simulink model "INS"  (R2018b)
settings: configuration reference "ins_config" (kept outside this file)
values from neighbouring files (symbols this model uses):
  INS_EXPORT = Simulink.Parameter(INS_EXPORT_VALUE)    [base_ins_init.m]    (also in ins_model_init.m)
  INS_PARAM = Simulink.Parameter(INS_PARAM_VALUE)    [base_ins_init.m]    (also in ins_model_init.m)
undefined symbols (not defined in the file or in its folder): DiscIntNeverNeededParam, INS_CONST
libraries: simulink x95, AP_Math x15, Filter x6, Quaternion x2, Rotation x2
(part 4 of 4)

== system INS/Data_Fusion/AHRS/Correct/Att_Correction/Attitude_Correct/Measured_Acc/OpticalFlow_Acc_Observer ==
  OptFlow_vel_O_mDs : Inport
  Enable : EnablePort  StatesWhenEnabling=reset
  Constant : Constant  Value=0  OutDataTypeStr=single
  ContinueLinearObserver : Subsystem  mask{wn=10, ksi=0.707}
      mask prompts: wn "Cut frequency (rad/s)"; ksi "Damping ratio"
  Mux : Mux  Inputs=2
  Reshape : Reshape  OutputDimensionality=Customize  OutputDimensions=[3,1]
  Selector : Selector  InputPortWidth=3  IndexOptions=Index vector (dialog)  Indices=[1 2]  OutputSizes=1
  Terminator : Terminator
  OptFlow_acc_O_mPs2 : Outport
  wires:
  Mux/1 -> Reshape/1
  OptFlow_vel_O_mDs/1 -> Selector/1
  Constant/1 -> Mux/2
  ContinueLinearObserver/2(x2) -> Mux/1
  ContinueLinearObserver/1(x1) -> Terminator/1
  Selector/1 -> ContinueLinearObserver/1(xr)
  Reshape/1 -> OptFlow_acc_O_mPs2/1

== system INS/Data_Fusion/AHRS/Correct/Att_Correction/Attitude_Correct/Measured_Acc/Routing ==
  gps_ob_enable : Inport
  GPS_acc_O_mPs2 : Inport  Port=2
  opt_flow_ob_enable : Inport  Port=3
  opt_flow_acc_O_mPs2 : Inport  Port=4
  GPS_Delay : Constant  Value=250/INS_EXPORT.period  OutDataTypeStr=uint16
  Logical Operator : Logic  Operator=OR  AllPortsSameDT=off  OutDataTypeStr=boolean
  Multiply{,1..3} (4 alike) : Product  OutDataTypeStr=single
  OptFlow_Delay : Constant  Value=50/INS_EXPORT.period  OutDataTypeStr=uint16
  Sum : Sum  Inputs=|++
  Sum1 : Sum  Inputs=|++
  Sum2 : Sum  Inputs=++|
  gravity : Constant  Value=[0;0;-INS_CONST.g]  VectorParams1D=off  OutDataTypeStr=single
  meas_acc_O_mPs2 : Outport
  acc_ob_valid : Outport  Port=2
  acc_delay : Outport  Port=3
  wires:
  gps_ob_enable/1 -> Logical Operator/1, Multiply/1, Multiply2/1
  Multiply2/1 -> Sum1/1
  GPS_Delay/1 -> Multiply2/2
  Multiply/1 -> Sum/1
  GPS_acc_O_mPs2/1 -> Multiply/2
  opt_flow_acc_O_mPs2/1 -> Multiply1/2
  opt_flow_ob_enable/1 -> Multiply1/1, Multiply3/1, Logical Operator/2
  Multiply1/1 -> Sum/2
  Logical Operator/1 -> acc_ob_valid/1
  OptFlow_Delay/1 -> Multiply3/2
  Sum1/1 -> acc_delay/1
  Multiply3/1 -> Sum1/2
  Sum2/1 -> meas_acc_O_mPs2/1
  Sum/1 -> Sum2/2
  gravity/1 -> Sum2/1

== system INS/Data_Fusion/Translation_Filter/CF/Bus_Assignment/Signal_Rounting/Meter_to_LatLon/Zero_Value_Exclusion ==
  u : Inport
  Abs : Abs
  Constant : Constant
  Product : Product  RndMeth=Zero
  Saturation : Saturate  UpperLimit=10e7  LowerLimit=thr
  Sign : Signum
  Switch : Switch  Criteria=u2 ~= 0
  y : Outport
  wires:
  u/1 -> Sign/1, Abs/1
  Abs/1 -> Saturation/1
  Saturation/1 -> Product/1
  Sign/1 -> Switch/2, Switch/1
  Product/1 -> y/1
  Switch/1 -> Product/2
  Constant/1 -> Switch/3

== system INS/Data_Fusion/Translation_Filter/CF/Horizontal_Filter/Correct/GPS_Correct/Holder ==
  in : Inport
  update : Inport  Port=2
  Gain3 : Gain  Gain=INS_CONST.dt  OutDataTypeStr=Inherit: Same as input
  Memory : Memory
  Switch : Switch  Criteria=u2 > Threshold
  out : Outport
  wires:
  update/1 -> Switch/2
  Switch/1 -> Memory/1, Gain3/1
  in/1 -> Switch/1
  Memory/1 -> Switch/3
  Gain3/1 -> out/1

== system INS/Data_Fusion/Translation_Filter/CF/Horizontal_Filter/Correct/GPS_Correct/Measurement ==
  X : Inport
  Processed_Data : Inport  Port=2
  Bus Selector : BusSelector  OutputSignals=Sensor_Meas.GPS_Meas.mue_rad,Sensor_Meas.GPS_Meas.lambda_rad,Init_Condition.WGS84_Ref.WGS84_pos_ref.mue_0_rad,Init_Condition.WGS84_Ref.WGS84_pos_ref.lambda_0_rad,Init_Condition.WGS84_Ref.WGS84_derivatives_ref.dx_dmue_0,Init_Condition.WGS84_Ref.WGS84_derivatives_ref.dy_dlambda_0
  Bus Selector1 : BusSelector  OutputSignals=Sensor_Meas.GPS_Meas.vel_N_mPs,Sensor_Meas.GPS_Meas.vel_E_mPs
  Data Type Conversion : DataTypeConversion  OutDataTypeStr=single
  Multiply : Product
  Mux{,1..4} (5 alike) : Mux  Inputs=2
  Remove_Bias : Subsystem
  Reshape3 : Reshape  OutputDimensionality=Customize  OutputDimensions=[4,1]
  Sum : Sum  Inputs=|+-
  Z : Outport
  bias_update : Outport  Port=2
  wires:
  X/1 -> Remove_Bias/2(X)
  Data Type Conversion/1 -> Remove_Bias/3(xy_meas_m)
  Remove_Bias/2(xy_O_m) -> Mux3/1
  Bus Selector1/2 -> Mux4/2  "<vel_E_mPs>"
  Bus Selector1/1 -> Mux4/1  "<vel_N_mPs>"
  Multiply/1 -> Data Type Conversion/1  "xy"
  Mux2/1 -> Multiply/2
  Sum/1 -> Multiply/1
  Bus Selector/6 -> Mux2/2  "<dy_dlambda_0>"
  Bus Selector/5 -> Mux2/1  "<dx_dmue_0>"
  Mux1/1 -> Sum/2
  Mux/1 -> Sum/1
  Bus Selector/4 -> Mux1/2  "<lambda_0_rad>"
  Bus Selector/3 -> Mux1/1  "<mue_0_rad>"
  Bus Selector/2 -> Mux/2  "<lambda_rad>"
  Bus Selector/1 -> Mux/1  "<mue_rad>"
  Processed_Data/1 -> Bus Selector/1, Bus Selector1/1, Remove_Bias/1(Processed_Data)
  Remove_Bias/1(bias_update) -> bias_update/1
  Mux3/1 -> Reshape3/1
  Reshape3/1 -> Z/1
  Mux4/1 -> Mux3/2

== system INS/Data_Fusion/Translation_Filter/CF/Horizontal_Filter/Correct/GPS_Correct/Observation ==
  X : Inport
  reset : Inport  Port=2
  Mux : Mux
  Reshape : Reshape  OutputDimensionality=Customize  OutputDimensions=[4,1]
  Selector : Selector  InputPortWidth=6  IndexOptions=Index vector (dialog)  Indices=[1]  OutputSizes=1
  Selector1 : Selector  InputPortWidth=6  IndexOptions=Index vector (dialog)  Indices=[2]  OutputSizes=1
  Selector2 : Selector  InputPortWidth=6  IndexOptions=Index vector (dialog)  Indices=[3]  OutputSizes=1
  Selector3 : Selector  InputPortWidth=6  IndexOptions=Index vector (dialog)  Indices=[4]  OutputSizes=1
  vn_delay : Delay  DelayLength=100/INS_EXPORT.period  InitialConditionSource=Input port  ExternalReset=Rising
      settings: InputPortMap=u0,r5,p4
  vn_delay1 : Delay  DelayLength=100/INS_EXPORT.period  InitialConditionSource=Input port  ExternalReset=Rising
      settings: InputPortMap=u0,r5,p4
  x_delay : Delay  DelayLength=150/INS_EXPORT.period  InitialConditionSource=Input port  ExternalReset=Rising
      settings: InputPortMap=u0,r5,p4
  x_delay1 : Delay  DelayLength=150/INS_EXPORT.period  InitialConditionSource=Input port  ExternalReset=Rising
      settings: InputPortMap=u0,r5,p4
  HX : Outport
  wires:
  Mux/1 -> Reshape/1
  Reshape/1 -> HX/1
  reset/1 -> vn_delay1/2, x_delay/2, x_delay1/2, vn_delay/2
  x_delay1/1 -> Mux/2
  vn_delay/1 -> Mux/3
  vn_delay1/1 -> Mux/4
  x_delay/1 -> Mux/1
  Selector/1 -> x_delay/3, x_delay/1
  X/1 -> Selector3/1, Selector2/1, Selector1/1, Selector/1
  Selector1/1 -> x_delay1/3, x_delay1/1
  Selector2/1 -> vn_delay/3, vn_delay/1
  Selector3/1 -> vn_delay1/3, vn_delay1/1

== system INS/Data_Fusion/Translation_Filter/CF/Horizontal_Filter/Correct/GPS_Correct/Scaling ==
  y : Inport
  Demux : Demux  Outputs=2
  Gain : Gain  Gain=2  OutDataTypeStr=single
  Gain1 : Gain  Commented=on  Gain=1.5  OutDataTypeStr=single
  Gain2 : Gain  Gain=-1  OutDataTypeStr=single
  Gain3 : Gain  Gain=0  OutDataTypeStr=single
  Mux : Mux  Inputs=3
  Reshape : Reshape  OutputDimensionality=Customize  OutputDimensions=[6,1]
  X_error : Outport
  wires:
  y/1 -> Demux/1
  Demux/1 -> Gain3/1
  Demux/2 -> Gain2/1, Gain/1
  Gain2/1 -> Mux/3
  Mux/1 -> Reshape/1
  Gain3/1 -> Mux/1
  Gain/1 -> Mux/2
  Reshape/1 -> X_error/1

== system INS/Data_Fusion/Translation_Filter/CF/Horizontal_Filter/Predict/Propagate/States_Init ==
  Processed_Data : Inport
  Constant : Constant  Value=[0;0]  VectorParams1D=off  OutDataTypeStr=single
  Mux : Mux  Inputs=3
  Pos_Init : Subsystem
  Vel_Init : Subsystem
  X_0 : Outport
  wires:
  Processed_Data/1 -> Pos_Init/1(Processed_Data), Vel_Init/1(Processed_Data)
  Constant/1 -> Mux/3  "ba_xy_0"
  Mux/1 -> X_0/1
  Vel_Init/1(vel_NE_0) -> Mux/2
  Pos_Init/1(XY_0) -> Mux/1

== system INS/Data_Fusion/Translation_Filter/CF/Verticle_Filter/Correct/Baro_Correct/Baro_Correct ==
  Processed_Data : Inport
  X_Predict : Inport  Port=2
  Enable : EnablePort  StatesWhenEnabling=reset
  Bus Selector : BusSelector  OutputSignals=Init_Condition.height_reset
  Bus Selector1 : BusSelector  OutputSignals=Sensor_Meas.Baro_Meas.timestamp_ms
  Detect Change : simulink/Logic and Bit Operations/Detect Change  vinit=0  OutDataTypeStr=boolean
  Holder : Subsystem
  Logical Operator : Logic  Operator=OR  AllPortsSameDT=off  OutDataTypeStr=boolean
  Measurement : Subsystem
  Observation : Subsystem
  Scaling : Subsystem  mask{w=0.707}
      mask prompts: w "omega"
  Sum : Sum  Inputs=|-+
  Sum1 : Sum  Inputs=++|
  X_Next : Outport
  wires:
  Observation/1(HX) -> Sum/1  "Baro_HX"
  Measurement/1(Z) -> Sum/2  "Baro_Z"
  Processed_Data/1 -> Bus Selector/1, Measurement/2(Processed_Data), Bus Selector1/1
  Sum/1 -> Scaling/1(y)  "baro_err"
  Bus Selector1/1 -> Detect Change/1  "<timestamp_ms>"
  Holder/1(out) -> Sum1/2
  Sum1/1 -> X_Next/1
  X_Predict/1 -> Measurement/1(X), Observation/1(X), Sum1/1
  Bus Selector/1 -> Observation/2(reset)  "<height_reset>"
  Logical Operator/1 -> Holder/2(update)
  Detect Change/1 -> Logical Operator/2
  Measurement/2(bias_update) -> Logical Operator/1
  Scaling/1(X_error) -> Holder/1(in)

== system INS/Data_Fusion/Translation_Filter/CF/Verticle_Filter/Correct/GPS_Correct/GPS_Correct ==
  Processed_Data : Inport
  X_Predict : Inport  Port=2
  Enable : EnablePort  StatesWhenEnabling=reset
  Bus Selector : BusSelector  OutputSignals=Init_Condition.height_reset
  Bus Selector1 : BusSelector  OutputSignals=Sensor_Meas.Baro_Meas.timestamp_ms
  Detect Change : simulink/Logic and Bit Operations/Detect Change  vinit=0  OutDataTypeStr=boolean
  Holder : Subsystem
  Logical Operator : Logic  Operator=OR  AllPortsSameDT=off  OutDataTypeStr=boolean
  Measurement : Subsystem
  Observation : Subsystem
  Scaling : Subsystem
  Sum : Sum  Inputs=|-+
  Sum1 : Sum  Inputs=++|
  X_Next : Outport
  wires:
  Observation/1(HX) -> Sum/1  "GPS_Z_HX"
  Measurement/1(Z) -> Sum/2  "GPS_Z_Z"
  Processed_Data/1 -> Bus Selector/1, Measurement/2(Processed_Data), Bus Selector1/1
  Sum/1 -> Scaling/1(y)
  Bus Selector1/1 -> Detect Change/1  "<timestamp_ms>"
  Holder/1(out) -> Sum1/2
  Sum1/1 -> X_Next/1
  X_Predict/1 -> Measurement/1(X), Observation/1(X), Sum1/1
  Bus Selector/1 -> Observation/2(reset)  "<height_reset>"
  Logical Operator/1 -> Holder/2(update)
  Detect Change/1 -> Logical Operator/2
  Measurement/2(bias_update) -> Logical Operator/1
  Scaling/1(X_error) -> Holder/1(in)

== system INS/Data_Fusion/Translation_Filter/CF/Verticle_Filter/Predict/Propagate/States_Init ==
  Processed_Data : Inport
  Baro_Height_Init : Subsystem
  Constant : Constant  Value=0  OutDataTypeStr=single
  GPS_Height_Init : Subsystem
  Merge : Merge  Inputs=3
  Merge1 : Merge  Inputs=3
  Mux : Mux  Inputs=3
  Sonar_Height_Init : Subsystem
  X_0 : Outport
  wires:
  Constant/1 -> Mux/3  "ba_z_0"
  Sonar_Height_Init/1(h_0) -> Merge/2
  Mux/1 -> X_0/1
  Processed_Data/1 -> Baro_Height_Init/1(Processed_Data), Sonar_Height_Init/1(Processed_Data), GPS_Height_Init/1(Processed_Data)
  Merge/1 -> Mux/1  "h_0"
  GPS_Height_Init/1(h_0) -> Merge/1
  Merge1/1 -> Mux/2  "vel_D_0"
  GPS_Height_Init/2(vel_D) -> Merge1/1
  Sonar_Height_Init/2(vel_D) -> Merge1/2
  Baro_Height_Init/1(h_0) -> Merge/3
  Baro_Height_Init/2(vel_D) -> Merge1/3

== system INS/Data_Fusion/Translation_Filter/Process/Process_Data/Init_Condition/Pos_Reset/Height_Reset ==
  Rotation_Data : Inport
  Validity : Inport  Port=2
  global_reset : Inport  Port=3
  Bus Selector : BusSelector  OutputSignals=h_R_valid
  Detect Rise Positive : simulink/Logic and Bit Operations/Detect Rise Positive  vinit=0  OutDataTypeStr=boolean
  Logical Operator2 : Logic  Operator=OR  AllPortsSameDT=off  OutDataTypeStr=boolean
  Terminator : Terminator
  height_reset : Outport
  wires:
  Validity/1 -> Bus Selector/1
  global_reset/1 -> Logical Operator2/2
  Rotation_Data/1 -> Terminator/1
  Logical Operator2/1 -> height_reset/1
  Detect Rise Positive/1 -> Logical Operator2/1
  Bus Selector/1 -> Detect Rise Positive/1  "<h_R_valid>"

== system INS/Data_Fusion/Translation_Filter/Process/Process_Data/Init_Condition/Pos_Reset/Position_Reset ==
  Rotation_Data : Inport
  Validity : Inport  Port=2
  global_reset : Inport  Port=3
  Bus Selector : BusSelector  OutputSignals=xy_R_valid
  Bus Selector1 : BusSelector  OutputSignals=standstill
  Detect Rise Positive : simulink/Logic and Bit Operations/Detect Rise Positive  vinit=0  OutDataTypeStr=boolean
  Logical Operator2 : Logic  Operator=OR  AllPortsSameDT=off  OutDataTypeStr=boolean
  Terminator : Terminator
  pos_reset : Outport
  wires:
  Bus Selector/1 -> Detect Rise Positive/1  "<xy_R_valid>"
  Detect Rise Positive/1 -> Logical Operator2/1
  Logical Operator2/1 -> pos_reset/1
  Rotation_Data/1 -> Bus Selector1/1
  global_reset/1 -> Logical Operator2/2
  Validity/1 -> Bus Selector/1
  Bus Selector1/1 -> Terminator/1  "<standstill>"

== system INS/Data_Fusion/Translation_Filter/Process/Process_Data/Init_Condition/WGS84_Reference/Bus_Assignment ==
  WGS84_pos_ref : Inport
  WGS84_dpos_ref : Inport  Port=2
  WGS84_hgt_ref : Inport  Port=3
  WGS84_dhgt_ref : Inport  Port=4
  Bus Creator : BusCreator  Inputs=2
  Bus Creator1 : BusCreator  Inputs=3
  Bus Creator2 : BusCreator  Inputs=3
  Demux : Demux  Outputs=2
  Demux1 : Demux  Outputs=2
  WGS84_Ref : Outport
  wires:
  Bus Creator/1 -> WGS84_Ref/1
  Demux/1 -> Bus Creator1/1  "dx_dmue_0"
  Demux1/1 -> Bus Creator2/1  "mue_0_rad"
  Demux/2 -> Bus Creator1/2  "dy_dlambda_0"
  Demux1/2 -> Bus Creator2/2  "lambda_0_rad"
  Bus Creator2/1 -> Bus Creator/2  "WGS84_pos_ref"
  WGS84_dhgt_ref/1 -> Bus Creator1/3  "dz_dh_0"
  WGS84_hgt_ref/1 -> Bus Creator2/3  "h_0_m"
  Bus Creator1/1 -> Bus Creator/1  "WGS84_derivatives_ref"
  WGS84_dpos_ref/1 -> Demux/1
  WGS84_pos_ref/1 -> Demux1/1

== system INS/Data_Fusion/Translation_Filter/Process/Process_Data/Init_Condition/WGS84_Reference/WGS84_Height_Ref ==
  WGS84_position : Inport
  Translation_Data : Inport  Port=2
  Validity : Inport  Port=3
  WGS84_derivatives : Inport  Port=4
  Bus Selector1 : BusSelector  OutputSignals=h_R_m
  Bus Selector2 : BusSelector  OutputSignals=altitude_valid
  Delay : Delay  DelayLength=1
  Delay1 : Delay  DelayLength=1
  Detect Rise Positive3 : simulink/Logic and Bit Operations/Detect Rise Positive  vinit=0  OutDataTypeStr=boolean
  Divide : Product  Inputs=*/
  Selector : Selector  InputPortWidth=3  IndexOptions=Index vector (dialog)  Indices=3  OutputSizes=1
  Selector1 : Selector  InputPortWidth=3  IndexOptions=Index vector (dialog)  Indices=3  OutputSizes=1
  Sum : Sum  Inputs=|+-
  Switch4 : Switch  Criteria=u2 > Threshold
  Switch5 : Switch  Criteria=u2 > Threshold
  WGS84_hgt_ref : Outport
  WGS84_dhgt_ref : Outport  Port=2
  wires:
  Delay1/1 -> Switch4/3
  Switch4/1 -> Delay1/1, WGS84_hgt_ref/1  "WGS84_pos_ref"
  Detect Rise Positive3/1 -> Switch5/2, Switch4/2
  Bus Selector2/1 -> Detect Rise Positive3/1  "<altitude_valid>"
  WGS84_derivatives/1 -> Selector/1
  Switch5/1 -> Delay/1, WGS84_dhgt_ref/1  "WGS84_derivatives_ref"
  Delay/1 -> Switch5/3
  Validity/1 -> Bus Selector2/1
  Translation_Data/1 -> Bus Selector1/1
  Sum/1 -> Switch4/1
  Bus Selector1/1 -> Divide/1  "<h_R_m>"
  Divide/1 -> Sum/2
  WGS84_position/1 -> Selector1/1
  Selector/1 -> Switch5/1, Divide/2
  Selector1/1 -> Sum/1

== system INS/Data_Fusion/Translation_Filter/Process/Process_Data/Init_Condition/WGS84_Reference/WGS84_Position_Ref ==
  WGS84_position : Inport
  Translation_Data : Inport  Port=2
  Validity : Inport  Port=3
  WGS84_derivatives : Inport  Port=4
  Bus Selector1 : BusSelector  OutputSignals=x_R_m,y_R_m
  Bus Selector2 : BusSelector  OutputSignals=lon_lat_valid
  Delay : Delay  DelayLength=1
  Delay1 : Delay  DelayLength=1
  Detect Rise Positive3 : simulink/Logic and Bit Operations/Detect Rise Positive  vinit=0  OutDataTypeStr=boolean
  Divide : Product  Inputs=*/
  Mux : Mux  Inputs=2
  Selector : Selector  InputPortWidth=3  IndexOptions=Index vector (dialog)  Indices=[1 2]  OutputSizes=1
  Selector1 : Selector  InputPortWidth=3  IndexOptions=Index vector (dialog)  Indices=[1 2]  OutputSizes=1
  Sum : Sum  Inputs=|+-
  Switch4 : Switch  Criteria=u2 > Threshold
  Switch5 : Switch  Criteria=u2 > Threshold
  WGS84_pos_ref : Outport
  WGS84_dpos_ref : Outport  Port=2
  wires:
  Delay/1 -> Switch4/3
  Bus Selector1/1 -> Mux/1  "<x_R_m>"
  Switch4/1 -> Delay/1, WGS84_pos_ref/1  "WGS84_pos_ref"
  Mux/1 -> Divide/1  "WGS84_pos_ref"
  Detect Rise Positive3/1 -> Switch4/2, Switch5/2
  Bus Selector2/1 -> Detect Rise Positive3/1  "<lon_lat_valid>"
  WGS84_derivatives/1 -> Selector/1
  Switch5/1 -> Delay1/1, WGS84_dpos_ref/1  "WGS84_derivatives_ref"
  Delay1/1 -> Switch5/3
  Validity/1 -> Bus Selector2/1
  Translation_Data/1 -> Bus Selector1/1
  Sum/1 -> Switch4/1
  Bus Selector1/2 -> Mux/2  "<y_R_m>"
  Divide/1 -> Sum/2
  WGS84_position/1 -> Selector1/1
  Selector/1 -> Switch5/1, Divide/2
  Selector1/1 -> Sum/1

== system INS/Data_Fusion/Translation_Filter/Process/Process_Data/Sensor_Valid/Position_Validity/Horizontal_Validity ==
  Sensor_Status : Inport
  Bus Selector : BusSelector  OutputSignals=GPS_Status.GPS_vaid,GPS_Status.pos_quality,OptFlow_Status.opt_flow_valid
  Compare To Zero : simulink/Logic and Bit Operations/Compare To Zero  relop=>  OutDataTypeStr=boolean
  Logical Operator : Logic  AllPortsSameDT=off  OutDataTypeStr=boolean
  Logical Operator1 : Logic  Operator=OR  AllPortsSameDT=off  OutDataTypeStr=boolean
  Signal Copy : SignalConversion  OverrideOpt=off
  Signal Copy1 : SignalConversion  OverrideOpt=off
  WGS84_pos_valid : Outport
  xy_R_valid : Outport  Port=2
  wires:
  Bus Selector/1 -> Logical Operator/1  "<GPS_vaid>"
  Logical Operator/1 -> Logical Operator1/1, Signal Copy/1
  Sensor_Status/1 -> Bus Selector/1
  Compare To Zero/1 -> Logical Operator/2
  Bus Selector/2 -> Compare To Zero/1  "<pos_quality>"
  Signal Copy/1 -> WGS84_pos_valid/1
  Signal Copy1/1 -> xy_R_valid/1
  Bus Selector/3 -> Logical Operator1/2  "<opt_flow_valid>"
  Logical Operator1/1 -> Signal Copy1/1

== system INS/Data_Fusion/Translation_Filter/Process/Process_Data/Sensor_Valid/Position_Validity/Vertical_Validity ==
  Sensor_Status : Inport
  Bus Selector : BusSelector  OutputSignals=GPS_Status.GPS_vaid,GPS_Status.pos_quality,Sonar_Status.sonar_valid,Baro_Status.baro_valid
  Compare To Zero : simulink/Logic and Bit Operations/Compare To Zero  relop=>  OutDataTypeStr=boolean
  Logical Operator : Logic  AllPortsSameDT=off  OutDataTypeStr=boolean
  Logical Operator2 : Logic  Operator=OR  Inputs=3  AllPortsSameDT=off  OutDataTypeStr=boolean
  WGS84_height_valid : Outport
  h_R_valid : Outport  Port=2
  wires:
  Bus Selector/2 -> Compare To Zero/1  "<pos_quality>"
  Compare To Zero/1 -> Logical Operator/2
  Logical Operator/1 -> Logical Operator2/1, WGS84_height_valid/1
  Sensor_Status/1 -> Bus Selector/1
  Logical Operator2/1 -> h_R_valid/1
  Bus Selector/1 -> Logical Operator/1  "<GPS_vaid>"
  Bus Selector/3 -> Logical Operator2/2  "<sonar_valid>"
  Bus Selector/4 -> Logical Operator2/3  "<baro_valid>"

== system INS/Data_Fusion/AHRS/Correct/Att_Correction/Attitude_Correct/Acc_Correct/Heading_Correct/Modulus ==
  x : Inport
  Dot Product : DotProduct  InputSameDT=on  OutDataTypeStr=Inherit: Inherit via internal rule
  Sqrt : Sqrt  SaturateOnIntegerOverflow=on
  mag_x : Outport
  wires:
  x/1 -> Dot Product/1, Dot Product/2
  Dot Product/1 -> Sqrt/1
  Sqrt/1 -> mag_x/1

== system INS/Data_Fusion/AHRS/Correct/Att_Correction/Attitude_Correct/Acc_Correct/Heading_Correct/Modulus1 ==
  x : Inport
  Dot Product : DotProduct  InputSameDT=on  OutDataTypeStr=Inherit: Inherit via internal rule
  Sqrt : Sqrt  SaturateOnIntegerOverflow=on
  mag_x : Outport
  wires:
  x/1 -> Dot Product/1, Dot Product/2
  Dot Product/1 -> Sqrt/1
  Sqrt/1 -> mag_x/1

== system INS/Data_Fusion/AHRS/Correct/Att_Correction/Attitude_Correct/Acc_Correct/Heading_Correct/Weight ==
  x1 : Inport
  x2 : Inport  Port=2
  Abs : Abs
  Constant : Constant  Value=0.1  OutDataTypeStr=Inherit: Inherit via back propagation
  Constant1 : Constant  Value=1.0  OutDataTypeStr=Inherit: Inherit via back propagation
  Divide : Product  Inputs=/*
  Gain : Gain  Gain=2
  Max : MinMax  Function=max  Inputs=2
  Max1 : MinMax  Function=max  Inputs=2
  Saturation : Saturate  UpperLimit=1.0  LowerLimit=0.0
  Subtract : Sum  Inputs=+-
  Subtract1 : Sum  Inputs=+-
  y : Outport
  wires:
  Subtract1/1 -> Saturation/1
  x2/1 -> Max/2, Subtract/2
  x1/1 -> Max/1, Subtract/1
  Subtract/1 -> Abs/1
  Abs/1 -> Gain/1
  Max/1 -> Max1/2
  Constant/1 -> Max1/1
  Gain/1 -> Divide/2
  Max1/1 -> Divide/1
  Constant1/1 -> Subtract1/1
  Divide/1 -> Subtract1/2
  Saturation/1 -> y/1

== system INS/Data_Fusion/AHRS/Correct/Att_Correction/Attitude_Correct/Acc_Correct/Verticle_Correct/Cross_Product2 ==
  a : Inport
  b : Inport  Port=2
  Column Vector : Reshape  OutputDimensionality=Column vector (2-D)
  Column Vector1 : Reshape  OutputDimensionality=Column vector (2-D)
  Column Vector2 : Reshape  OutputDimensionality=Column vector (2-D)
  Data Type Duplicate : DataTypeDuplicate  NumInputPorts=3
  Demux : Demux  Outputs=3
  Demux1 : Demux  Outputs=3
  Mux : Mux  Inputs=3
  Product{,1..5} (6 alike) : Product  RndMeth=Zero
  Subtract : Sum  Inputs=+-
  Subtract1 : Sum  Inputs=+-
  Subtract2 : Sum  Inputs=+-
  axb : Outport
  wires:
  a/1 -> Data Type Duplicate/3, Column Vector1/1
  Column Vector1/1 -> Demux/1
  Column Vector2/1 -> Demux1/1
  b/1 -> Data Type Duplicate/2, Column Vector2/1
  Demux/2 -> Product5/1, Product/1
  Demux1/3 -> Product/2, Product3/2
  Product/1 -> Subtract/1
  Product1/1 -> Subtract/2
  Demux/3 -> Product1/1, Product2/1
  Demux1/2 -> Product1/2, Product4/2
  Product2/1 -> Subtract1/1
  Product3/1 -> Subtract1/2
  Demux1/1 -> Product2/2, Product5/2
  Demux/1 -> Product4/1, Product3/1
  Product4/1 -> Subtract2/1
  Product5/1 -> Subtract2/2
  Subtract/1 -> Mux/1
  Subtract1/1 -> Mux/2
  Subtract2/1 -> Mux/3
  Mux/1 -> Column Vector/1
  Column Vector/1 -> Data Type Duplicate/1, axb/1

== system INS/Data_Fusion/AHRS/Correct/Att_Correction/Attitude_Correct/Acc_Correct/Verticle_Correct/NonlinerSaturation ==
  u : Inport
  lim : Inport  Port=2
  Constant1 : Constant  Value=1e-3  OutDataTypeStr=Inherit: Inherit via back propagation
  Divide : Product  Inputs=**/
  Divide1 : Product  Inputs=*/
  Divide2 : Product  Inputs=**
  MinMax : MinMax  Function=max  Inputs=2
  Saturation : Saturate  UpperLimit=pi/2  LowerLimit=-pi/2
  Trigonometric Function : Trigonometry
  vec_modulus : AP_Math/vec_modulus  SystemSampleTime=-1
  y : Outport
  wires:
  Constant1/1 -> MinMax/2
  Saturation/1 -> Trigonometric Function/1
  u/1 -> vec_modulus/1, Divide/1
  Trigonometric Function/1 -> Divide2/1
  Divide/1 -> y/1
  vec_modulus/1 -> Divide1/1, MinMax/1
  Divide1/1 -> Saturation/1
  Divide2/1 -> Divide/2
  lim/1 -> Divide1/2, Divide2/2
  MinMax/1 -> Divide/3

== system INS/Data_Fusion/AHRS/Correct/Att_Correction/Attitude_Correct/Measured_Acc/GPS_Acc_Observer/ContinueLinearObserver ==
  xr : Inport
  reset : Inport  Port=2
  Add : Sum
  Discrete-Time Integrator : DiscreteIntegrator  ExternalReset=level  SampleTime=-1  ICPrevOutput=DiscIntNeverNeededParam  ICPrevScaledInput=DiscIntNeverNeededParam
  Discrete-Time Integrator1 : DiscreteIntegrator  ExternalReset=level  InitialConditionSource=external  SampleTime=-1  ICPrevOutput=DiscIntNeverNeededParam  ICPrevScaledInput=DiscIntNeverNeededParam
  Gain2 : Gain  Gain=2*ksi*wn
  Gain3 : Gain  Gain=wn^2
  Subtract : Sum  Inputs=+-
  x1 : Outport
  x2 : Outport  Port=2
  wires:
  Gain3/1 -> Discrete-Time Integrator/1
  xr/1 -> Discrete-Time Integrator1/3, Subtract/1
  Discrete-Time Integrator1/1 -> Subtract/2, x1/1
  Add/1 -> Discrete-Time Integrator1/1
  Subtract/1 -> Gain2/1, Gain3/1
  Discrete-Time Integrator/1 -> x2/1, Add/2
  Gain2/1 -> Add/1
  reset/1 -> Discrete-Time Integrator1/2, Discrete-Time Integrator/2

== system INS/Data_Fusion/AHRS/Correct/Att_Correction/Attitude_Correct/Measured_Acc/OpticalFlow_Acc_Observer/ContinueLinearObserver ==
  xr : Inport
  Add : Sum
  Discrete-Time Integrator : DiscreteIntegrator  InitialConditionSource=external  SampleTime=-1  ICPrevOutput=DiscIntNeverNeededParam  ICPrevScaledInput=DiscIntNeverNeededParam
  Discrete-Time Integrator1 : DiscreteIntegrator  SampleTime=-1  ICPrevOutput=DiscIntNeverNeededParam  ICPrevScaledInput=DiscIntNeverNeededParam
  Gain2 : Gain  Gain=2*ksi*wn
  Gain3 : Gain  Gain=wn^2
  Subtract : Sum  Inputs=+-
  x1 : Outport
  x2 : Outport  Port=2
  wires:
  Gain2/1 -> Add/1
  Discrete-Time Integrator/1 -> x2/1, Add/2
  Subtract/1 -> Gain3/1, Gain2/1
  Add/1 -> Discrete-Time Integrator1/1
  Discrete-Time Integrator1/1 -> x1/1, Subtract/2
  xr/1 -> Subtract/1, Discrete-Time Integrator/2
  Gain3/1 -> Discrete-Time Integrator/1

== system INS/Data_Fusion/Translation_Filter/CF/Horizontal_Filter/Correct/GPS_Correct/Measurement/Remove_Bias ==
  Processed_Data : Inport
  X : Inport  Port=2
  xy_meas_m : Inport  Port=3
  Pos_Error_Bias : Subsystem
  Sum1 : Sum  Inputs=|++
  bias_update : Outport
  xy_O_m : Outport  Port=2
  wires:
  Processed_Data/1 -> Pos_Error_Bias/3(Processed_Data)
  X/1 -> Pos_Error_Bias/2(X)
  Sum1/1 -> xy_O_m/1
  Pos_Error_Bias/1(bias) -> Sum1/2
  xy_meas_m/1 -> Sum1/1, Pos_Error_Bias/1(xy_meas_m)  "gps_xy_m"
  Pos_Error_Bias/2(bias_update) -> bias_update/1

== system INS/Data_Fusion/Translation_Filter/CF/Horizontal_Filter/Predict/Propagate/States_Init/Pos_Init ==
  Processed_Data : Inport
  Bus Selector : BusSelector  OutputSignals=Sensor_Status.GPS_Status.GPS_vaid
  GPS_Pos_Init : Subsystem
  XY_0 : Outport
  wires:
  Processed_Data/1 -> GPS_Pos_Init/1(Processed_Data), Bus Selector/1
  GPS_Pos_Init/1(X_0) -> XY_0/1  "xy_0"
  Bus Selector/1 -> GPS_Pos_Init/Enable  "<GPS_vaid>"

== system INS/Data_Fusion/Translation_Filter/CF/Horizontal_Filter/Predict/Propagate/States_Init/Vel_Init ==
  Processed_Data : Inport
  Bus Selector : BusSelector  OutputSignals=Sensor_Status.GPS_Status.GPS_vaid
  GPS_Vel_Init : Subsystem
  Logical Operator : Logic  Operator=NOT  AllPortsSameDT=off  OutDataTypeStr=boolean
  Merge1 : Merge
  OptFlow_Vel_Init : Subsystem
  vel_NE_0 : Outport
  wires:
  GPS_Vel_Init/1(Vel_NE_0) -> Merge1/1
  Processed_Data/1 -> GPS_Vel_Init/1(Processed_Data), OptFlow_Vel_Init/1(Processed_Data), Bus Selector/1
  OptFlow_Vel_Init/1(Vel_NE_0) -> Merge1/2
  Merge1/1 -> vel_NE_0/1  "vel_NE_0"
  Bus Selector/1 -> Logical Operator/1, GPS_Vel_Init/Enable  "<GPS_vaid>"
  Logical Operator/1 -> OptFlow_Vel_Init/Enable

== system INS/Data_Fusion/Translation_Filter/CF/Verticle_Filter/Correct/Baro_Correct/Baro_Correct/Holder ==
  in : Inport
  update : Inport  Port=2
  Delay : Delay  DelayLength=1
  Gain : Gain  Gain=INS_CONST.dt  OutDataTypeStr=Inherit: Same as input
  Switch : Switch  Criteria=u2 > Threshold
  out : Outport
  wires:
  update/1 -> Switch/2
  Switch/1 -> Delay/1, Gain/1
  in/1 -> Switch/1
  Delay/1 -> Switch/3
  Gain/1 -> out/1

== system INS/Data_Fusion/Translation_Filter/CF/Verticle_Filter/Correct/Baro_Correct/Baro_Correct/Measurement ==
  X : Inport
  Processed_Data : Inport  Port=2
  Bias_Estimate : Subsystem
  Bus Selector : BusSelector  OutputSignals=Sensor_Meas.Baro_Meas.h_R_m
  Sum1 : Sum  Inputs=|++
  Z : Outport
  bias_update : Outport  Port=2
  wires:
  Bus Selector/1 -> Bias_Estimate/1(h_m), Sum1/1  "<h_R_m>"
  Bias_Estimate/1(bias) -> Sum1/2
  X/1 -> Bias_Estimate/3(X)
  Processed_Data/1 -> Bias_Estimate/2(Processed_Data), Bus Selector/1
  Sum1/1 -> Z/1
  Bias_Estimate/2(bias_update) -> bias_update/1

== system INS/Data_Fusion/Translation_Filter/CF/Verticle_Filter/Correct/Baro_Correct/Baro_Correct/Observation ==
  note: Delay compensate due to sensor
      | measurement delay
  X : Inport
  reset : Inport  Port=2
  Selector : Selector  InputPortWidth=3  IndexOptions=Index vector (dialog)  Indices=[1]  OutputSizes=1
  x_delay : Delay  DelayLength=20/INS_EXPORT.period  InitialConditionSource=Input port  ExternalReset=Rising
      settings: InputPortMap=u0,r5,p4
  HX : Outport
  wires:
  reset/1 -> x_delay/2
  Selector/1 -> x_delay/1, x_delay/3  "HX"
  X/1 -> Selector/1
  x_delay/1 -> HX/1

== system INS/Data_Fusion/Translation_Filter/CF/Verticle_Filter/Correct/Baro_Correct/Baro_Correct/Scaling ==
  y : Inport
  Gain : Gain  Gain=w^3
  Gain1 : Gain  Gain=-3*w^2
  Gain2 : Gain  Gain=3*w
  Mux : Mux  Inputs=3
  X_error : Outport
  wires:
  y/1 -> Gain/1, Gain2/1, Gain1/1
  Gain2/1 -> Mux/1
  Gain1/1 -> Mux/2
  Gain/1 -> Mux/3
  Mux/1 -> X_error/1

== system INS/Data_Fusion/Translation_Filter/CF/Verticle_Filter/Correct/GPS_Correct/GPS_Correct/Holder ==
  in : Inport
  update : Inport  Port=2
  Gain3 : Gain  Gain=INS_CONST.dt  OutDataTypeStr=Inherit: Same as input
  Memory : Memory
  Switch : Switch  Criteria=u2 > Threshold
  out : Outport
  wires:
  update/1 -> Switch/2
  Switch/1 -> Memory/1, Gain3/1
  in/1 -> Switch/1
  Memory/1 -> Switch/3
  Gain3/1 -> out/1

== system INS/Data_Fusion/Translation_Filter/CF/Verticle_Filter/Correct/GPS_Correct/GPS_Correct/Measurement ==
  X : Inport
  Processed_Data : Inport  Port=2
  Bus Selector : BusSelector  OutputSignals=Sensor_Meas.GPS_Meas.h_m,Init_Condition.WGS84_Ref.WGS84_pos_ref.h_0_m
  Bus Selector1 : BusSelector  OutputSignals=Sensor_Meas.GPS_Meas.vel_D_mPs
  Data Type Conversion : DataTypeConversion  OutDataTypeStr=single
  Mux : Mux  Inputs=2
  Pos_Error_Bias : Subsystem
  Sum : Sum  Inputs=|+-
  Sum1 : Sum  Inputs=|++
  Z : Outport
  bias_update : Outport  Port=2
  wires:
  Data Type Conversion/1 -> Sum1/1, Pos_Error_Bias/1(h_m)  "GPS_KFV_Z2"
  Bus Selector/2 -> Sum/2  "<h_0_m>"
  Bus Selector/1 -> Sum/1  "<h_m>"
  Processed_Data/1 -> Pos_Error_Bias/3(Processed_Data), Bus Selector1/1, Bus Selector/1
  Sum/1 -> Data Type Conversion/1
  X/1 -> Pos_Error_Bias/2(X)
  Sum1/1 -> Mux/1
  Pos_Error_Bias/1(bias) -> Sum1/2
  Pos_Error_Bias/2(bias_update) -> bias_update/1
  Bus Selector1/1 -> Mux/2  "<vel_D_mPs>"
  Mux/1 -> Z/1

== system INS/Data_Fusion/Translation_Filter/CF/Verticle_Filter/Correct/GPS_Correct/GPS_Correct/Observation ==
  X : Inport
  reset : Inport  Port=2
  Mux : Mux  Inputs=2
  Reshape : Reshape  OutputDimensionality=Customize  OutputDimensions=[2,1]
  Selector : Selector  InputPortWidth=3  IndexOptions=Index vector (dialog)  Indices=[1]  OutputSizes=1
  Selector1 : Selector  InputPortWidth=3  IndexOptions=Index vector (dialog)  Indices=[2]  OutputSizes=1
  h_delay : Delay  DelayLength=150/INS_EXPORT.period  InitialConditionSource=Input port  ExternalReset=Rising
      settings: InputPortMap=u0,r5,p4
  vd_delay : Delay  DelayLength=100/INS_EXPORT.period  InitialConditionSource=Input port  ExternalReset=Rising
      settings: InputPortMap=u0,r5,p4
  HX : Outport
  wires:
  reset/1 -> h_delay/2, vd_delay/2
  h_delay/1 -> Mux/1
  vd_delay/1 -> Mux/2
  Reshape/1 -> HX/1
  Mux/1 -> Reshape/1
  Selector/1 -> h_delay/3, h_delay/1
  X/1 -> Selector1/1, Selector/1
  Selector1/1 -> vd_delay/3, vd_delay/1

== system INS/Data_Fusion/Translation_Filter/CF/Verticle_Filter/Correct/GPS_Correct/GPS_Correct/Scaling ==
  y : Inport
  Demux : Demux  Outputs=2
  Gain : Gain  Gain=2  OutDataTypeStr=single
  Gain1 : Gain  Gain=0  OutDataTypeStr=single
  Gain2 : Gain  Gain=-1  OutDataTypeStr=single
  Gain3 : Gain  Commented=on  Gain=1.5  OutDataTypeStr=single
  Mux : Mux  Inputs=3
  X_error : Outport
  wires:
  y/1 -> Demux/1
  Demux/1 -> Gain1/1
  Demux/2 -> Gain2/1, Gain/1
  Gain2/1 -> Mux/3
  Mux/1 -> X_error/1
  Gain1/1 -> Mux/1
  Gain/1 -> Mux/2

== system INS/Data_Fusion/Translation_Filter/CF/Verticle_Filter/Predict/Propagate/States_Init/Baro_Height_Init ==
  Processed_Data : Inport
  Bus Selector : BusSelector  OutputSignals=Sensor_Enable.baro_enable
  Reference_Height : Subsystem
  h_0 : Outport
  vel_D : Outport  Port=2
  wires:
  Processed_Data/1 -> Bus Selector/1, Reference_Height/1(Processed_Data)
  Reference_Height/1(h_R_m) -> h_0/1  "h_0"
  Bus Selector/1 -> Reference_Height/Enable  "<baro_enable>"
  Reference_Height/2(vel_D_mDs) -> vel_D/1

== system INS/Data_Fusion/Translation_Filter/CF/Verticle_Filter/Predict/Propagate/States_Init/GPS_Height_Init ==
  Processed_Data : Inport
  Bus Selector : BusSelector  OutputSignals=Sensor_Enable.gps_height_enable
  Reference_Height : Subsystem
  h_0 : Outport
  vel_D : Outport  Port=2
  wires:
  Processed_Data/1 -> Bus Selector/1, Reference_Height/1(Processed_Data)
  Reference_Height/1(h_R_m) -> h_0/1  "h_0"
  Bus Selector/1 -> Reference_Height/Enable  "<gps_height_enable>"
  Reference_Height/2(vel_D_mDs) -> vel_D/1

== system INS/Data_Fusion/Translation_Filter/CF/Verticle_Filter/Predict/Propagate/States_Init/Sonar_Height_Init ==
  Processed_Data : Inport
  Bus Selector : BusSelector  OutputSignals=Sensor_Enable.sonar_enable
  Reference_Height : Subsystem
  h_0 : Outport
  vel_D : Outport  Port=2
  wires:
  Processed_Data/1 -> Bus Selector/1, Reference_Height/1(Processed_Data)
  Reference_Height/1(h_R_m) -> h_0/1  "h_0"
  Bus Selector/1 -> Reference_Height/Enable  "<sonar_enable>"
  Reference_Height/2(vel_D_mDs) -> vel_D/1

== system INS/Data_Fusion/Translation_Filter/CF/Horizontal_Filter/Correct/GPS_Correct/Measurement/Remove_Bias/Pos_Error_Bias ==
  xy_meas_m : Inport
  X : Inport  Port=2
  Processed_Data : Inport  Port=3
  Bias_Update : Subsystem
  Bus Selector1 : BusSelector  OutputSignals=Sensor_Enable.gps_enable
  Detect Increase : simulink/Logic and Bit Operations/Detect Increase  vinit=0.0  OutDataTypeStr=boolean
  Memory : Memory  InitialCondition=[0;0]
  Selector : Selector  InputPortWidth=6  IndexOptions=Index vector (dialog)  Indices=[1 2]  OutputSizes=1
  Switch : Switch  Criteria=u2 > Threshold  OutDataTypeStr=single
  bias : Outport
  bias_update : Outport  Port=2
  wires:
  xy_meas_m/1 -> Bias_Update/2(xy_meas_m)
  Processed_Data/1 -> Bus Selector1/1
  Detect Increase/1 -> bias_update/1, Switch/2
  Bus Selector1/1 -> Detect Increase/1  "<gps_enable>"
  Selector/1 -> Bias_Update/1(xy_est_m)  "gps_xy_est"
  Switch/1 -> bias/1, Memory/1  "gps_pos_bias"
  Bias_Update/1(bias) -> Switch/1
  X/1 -> Selector/1
  Memory/1 -> Switch/3

== system INS/Data_Fusion/Translation_Filter/CF/Horizontal_Filter/Predict/Propagate/States_Init/Pos_Init/GPS_Pos_Init ==
  Processed_Data : Inport
  Enable : EnablePort
  Bus Selector : BusSelector  OutputSignals=Sensor_Meas.GPS_Meas.mue_rad,Sensor_Meas.GPS_Meas.lambda_rad,Init_Condition.WGS84_Ref.WGS84_pos_ref.mue_0_rad,Init_Condition.WGS84_Ref.WGS84_pos_ref.lambda_0_rad,Init_Condition.WGS84_Ref.WGS84_derivatives_ref.dx_dmue_0,Init_Condition.WGS84_Ref.WGS84_derivatives_ref.dy_dlambda_0
  Data Type Conversion : DataTypeConversion  OutDataTypeStr=single
  Multiply : Product
  Mux1 : Mux  Inputs=2
  Mux2 : Mux  Inputs=2
  Mux3 : Mux  Inputs=2
  Sum : Sum  Inputs=|+-
  X_0 : Outport
  wires:
  Data Type Conversion/1 -> X_0/1
  Bus Selector/1 -> Mux1/1  "<mue_rad>"
  Mux3/1 -> Multiply/2
  Bus Selector/3 -> Mux2/1  "<mue_0_rad>"
  Bus Selector/4 -> Mux2/2  "<lambda_0_rad>"
  Mux2/1 -> Sum/2
  Bus Selector/6 -> Mux3/2  "<dy_dlambda_0>"
  Mux1/1 -> Sum/1
  Sum/1 -> Multiply/1
  Bus Selector/5 -> Mux3/1  "<dx_dmue_0>"
  Bus Selector/2 -> Mux1/2  "<lambda_rad>"
  Processed_Data/1 -> Bus Selector/1
  Multiply/1 -> Data Type Conversion/1  "xy_R_m"

== system INS/Data_Fusion/Translation_Filter/CF/Horizontal_Filter/Predict/Propagate/States_Init/Vel_Init/GPS_Vel_Init ==
  Processed_Data : Inport
  Enable : EnablePort
  Bus Selector : BusSelector  OutputSignals=Sensor_Meas.GPS_Meas.vel_N_mPs,Sensor_Meas.GPS_Meas.vel_E_mPs
  Mux : Mux  Inputs=2
  Reshape : Reshape  OutputDimensionality=Customize  OutputDimensions=[2,1]
  Vel_NE_0 : Outport
  wires:
  Mux/1 -> Reshape/1
  Reshape/1 -> Vel_NE_0/1
  Bus Selector/2 -> Mux/2  "<vel_E_mPs>"
  Bus Selector/1 -> Mux/1  "<vel_N_mPs>"
  Processed_Data/1 -> Bus Selector/1

== system INS/Data_Fusion/Translation_Filter/CF/Horizontal_Filter/Predict/Propagate/States_Init/Vel_Init/OptFlow_Vel_Init ==
  Processed_Data : Inport
  Enable : EnablePort
  Bus Selector : BusSelector  OutputSignals=Sensor_Meas.OptFlow_Meas.vel_x_O,Sensor_Meas.OptFlow_Meas.vel_y_O
  Mux : Mux  Inputs=2
  Reshape : Reshape  OutputDimensionality=Customize  OutputDimensions=[2,1]
  Vel_NE_0 : Outport
  wires:
  Reshape/1 -> Vel_NE_0/1
  Mux/1 -> Reshape/1
  Bus Selector/2 -> Mux/2  "<vel_y_O>"
  Bus Selector/1 -> Mux/1  "<vel_x_O>"
  Processed_Data/1 -> Bus Selector/1

== system INS/Data_Fusion/Translation_Filter/CF/Verticle_Filter/Correct/Baro_Correct/Baro_Correct/Measurement/Bias_Estimate ==
  h_m : Inport
  Processed_Data : Inport  Port=2
  X : Inport  Port=3
  Bias_Update : Subsystem
  Bus Selector1 : BusSelector  OutputSignals=Sensor_Enable.baro_enable
  Delay : Delay  DelayLength=1
  Detect Increase : simulink/Logic and Bit Operations/Detect Increase  vinit=0.0  OutDataTypeStr=boolean
  Selector : Selector  InputPortWidth=3  IndexOptions=Index vector (dialog)  Indices=1  OutputSizes=1
  Switch : Switch  Criteria=u2 > Threshold  OutDataTypeStr=single
  bias : Outport
  bias_update : Outport  Port=2
  wires:
  Delay/1 -> Switch/3
  X/1 -> Selector/1
  Bias_Update/1(bias) -> Switch/1
  Switch/1 -> Delay/1, bias/1  "baro_alt_bias"
  Selector/1 -> Bias_Update/1(height_est_m)
  h_m/1 -> Bias_Update/2(height_meas_m)
  Bus Selector1/1 -> Detect Increase/1  "<baro_enable>"
  Processed_Data/1 -> Bus Selector1/1
  Detect Increase/1 -> bias_update/1, Switch/2  "baro_bias_update"

== system INS/Data_Fusion/Translation_Filter/CF/Verticle_Filter/Correct/GPS_Correct/GPS_Correct/Measurement/Pos_Error_Bias ==
  h_m : Inport
  X : Inport  Port=2
  Processed_Data : Inport  Port=3
  Bias_Update : Subsystem
  Bus Selector1 : BusSelector  OutputSignals=Sensor_Enable.gps_height_enable
  Detect Increase : simulink/Logic and Bit Operations/Detect Increase  vinit=0.0  OutDataTypeStr=boolean
  Memory : Memory
  Selector : Selector  InputPortWidth=3  IndexOptions=Index vector (dialog)  Indices=1  OutputSizes=1
  Switch : Switch  Criteria=u2 > Threshold  OutDataTypeStr=single
  bias : Outport
  bias_update : Outport  Port=2
  wires:
  Memory/1 -> Switch/3
  X/1 -> Selector/1
  Bias_Update/1(bias) -> Switch/1
  Switch/1 -> Memory/1, bias/1  "gps_height_bias"
  Selector/1 -> Bias_Update/1(h_est_m)  "h_est_m1"
  Bus Selector1/1 -> Detect Increase/1  "<gps_height_enable>"
  Detect Increase/1 -> bias_update/1, Switch/2
  Processed_Data/1 -> Bus Selector1/1
  h_m/1 -> Bias_Update/2(h_meas_m)  "gps_h_meas"

== system INS/Data_Fusion/Translation_Filter/CF/Verticle_Filter/Predict/Propagate/States_Init/Baro_Height_Init/Reference_Height ==
  Processed_Data : Inport
  Enable : EnablePort
  Bus Selector : BusSelector  OutputSignals=Sensor_Meas.Baro_Meas.h_R_m
  Constant : Constant  Value=0  OutDataTypeStr=single
  Data Type Conversion : DataTypeConversion  OutDataTypeStr=single
  h_R_m : Outport
  vel_D_mDs : Outport  Port=2
  wires:
  Data Type Conversion/1 -> h_R_m/1
  Bus Selector/1 -> Data Type Conversion/1  "<h_R_m>"
  Processed_Data/1 -> Bus Selector/1
  Constant/1 -> vel_D_mDs/1

== system INS/Data_Fusion/Translation_Filter/CF/Verticle_Filter/Predict/Propagate/States_Init/GPS_Height_Init/Reference_Height ==
  Processed_Data : Inport
  Enable : EnablePort
  Bus Selector : BusSelector  OutputSignals=Sensor_Meas.GPS_Meas.h_m,Init_Condition.WGS84_Ref.WGS84_pos_ref.h_0_m,Sensor_Meas.GPS_Meas.vel_D_mPs
  Data Type Conversion : DataTypeConversion  OutDataTypeStr=single
  Data Type Conversion1 : DataTypeConversion  OutDataTypeStr=single
  Sum : Sum  Inputs=|+-
  h_R_m : Outport
  vel_D_mDs : Outport  Port=2
  wires:
  Data Type Conversion/1 -> h_R_m/1
  Bus Selector/2 -> Sum/2  "<h_0_m>"
  Bus Selector/1 -> Sum/1  "<h_m>"
  Processed_Data/1 -> Bus Selector/1
  Sum/1 -> Data Type Conversion/1  "h_R_m"
  Bus Selector/3 -> Data Type Conversion1/1  "<vel_D_mPs>"
  Data Type Conversion1/1 -> vel_D_mDs/1

== system INS/Data_Fusion/Translation_Filter/CF/Verticle_Filter/Predict/Propagate/States_Init/Sonar_Height_Init/Reference_Height ==
  Processed_Data : Inport
  Enable : EnablePort
  Bus Selector : BusSelector  OutputSignals=Sensor_Meas.Sonar_Meas.distance_m
  Constant : Constant  Value=0  OutDataTypeStr=single
  Data Type Conversion : DataTypeConversion  OutDataTypeStr=single
  h_R_m : Outport
  vel_D_mDs : Outport  Port=2
  wires:
  Data Type Conversion/1 -> h_R_m/1
  Bus Selector/1 -> Data Type Conversion/1  "<distance_m>"
  Processed_Data/1 -> Bus Selector/1
  Constant/1 -> vel_D_mDs/1

== system INS/Data_Fusion/Translation_Filter/CF/Horizontal_Filter/Correct/GPS_Correct/Measurement/Remove_Bias/Pos_Error_Bias/Bias_Update ==
  xy_est_m : Inport
  xy_meas_m : Inport  Port=2
  Sum : Sum  Inputs=+-|
  bias : Outport
  wires:
  xy_est_m/1 -> Sum/1
  xy_meas_m/1 -> Sum/2
  Sum/1 -> bias/1

== system INS/Data_Fusion/Translation_Filter/CF/Verticle_Filter/Correct/Baro_Correct/Baro_Correct/Measurement/Bias_Estimate/Bias_Update ==
  height_est_m : Inport
  height_meas_m : Inport  Port=2
  Sum : Sum  Inputs=+-|
  bias : Outport
  wires:
  Sum/1 -> bias/1
  height_meas_m/1 -> Sum/2  "height_meas_m"
  height_est_m/1 -> Sum/1  "height_est_m"

== system INS/Data_Fusion/Translation_Filter/CF/Verticle_Filter/Correct/GPS_Correct/GPS_Correct/Measurement/Pos_Error_Bias/Bias_Update ==
  h_est_m : Inport
  h_meas_m : Inport  Port=2
  Sum : Sum  Inputs=+-|
  bias : Outport
  wires:
  Sum/1 -> bias/1
  h_meas_m/1 -> Sum/2
  h_est_m/1 -> Sum/1
